simulink model "SM_INV_2L_ACCPR_PLL_DVC"  (R2019b)
settings: Solver=VariableStepAuto  StartTime=0.0  StopTime=simtime  FixedStep=1e-5  RelTol=1e-3
undefined symbols (not defined in the file or in its folder): plecs
settings Model: Creator=zya-wgo  LastModifiedBy=Jiani
settings DataIOCC: ReturnWorkspaceOutputs=off
settings DebuggingCC: MaxConsecutiveZCsMsg=warning  ArithmeticOperatorsInVariantConditions=warning
settings SFSimCC: SimUseLocalCustomCode=off  CustomCodeUndefinedFunction=UseInterfaceOnly
settings RTWCC: RTWUseLocalCustomCode=off

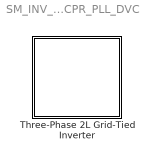
== system SM_INV_2L_ACCPR_PLL_DVC ==
  " Three-Phase 2L Grid-Tied Inverter" : Subsystem  LoadFcn=plecs('sl', 200);  InitFcn=plecs('sl', 214);  StartFcn=plecs('sl', 208);  StopFcn=plecs('sl', 209);  mask(PlecsCircuit){PLECSData=<binary blob, 15892 chars, not shown>}
      mask prompts: PLECSData "PLECS Data (Do not delete or modify!)"
      mask init:
      | % PLACE CUSTOM INITIALIZATIONS ABOVE
      | % DO NOT REMOVE
      | plecs('sl', 215);
      | % DO NOT REMOVE
      settings: CopyFcn=plecs('sl', 203);  DeleteFcn=plecs('sl', 205);  UndoDeleteFcn=plecs('sl', 206);  PreSaveFcn=plecs('sl', 211);  PostSaveFcn=plecs('sl', 201);  NameChangeFcn=plecs('sl', 210);  DestroyFcn=plecs('sl', 207);  PreCopyFcn=plecs('sl', 216);  OpenFcn=plecs('sl', 202);  ErrorFcn=plerrorfcn
      mask Help: web(['file:///' fullfile(plecsdoc, 'creatingacircuit.html')])
      mask Display: disp('PLECS\nCircuit')

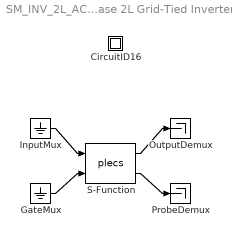
== system SM_INV_2L_ACCPR_PLL_DVC/ Three-Phase 2L Grid-Tied Inverter ==
  " CircuitID16 " : Subsystem
  " GateMux " : Ground
  " InputMux " : Ground
  " OutputDemux " : Terminator
  " ProbeDemux " : Terminator
  " S-Function " : S-Function  FunctionName=plecs  SFunctionDeploymentMode=off  EnableBusSupport=off
  wires:
  " InputMux "/1 -> " S-Function "/1
  " GateMux "/1 -> " S-Function "/2
  " S-Function "/1 -> " OutputDemux "/1
  " S-Function "/2 -> " ProbeDemux "/1

== system SM_INV_2L_ACCPR_PLL_DVC/ Three-Phase 2L Grid-Tied Inverter/ CircuitID16  ==
